simulink model "novel_topology_1"  (R2020a)
settings: Solver=FixedStepDiscrete  StartTime=0.0  StopTime=0.2  RelTol=1e-3
InitFcn:
  | novel_topology_1_param
values from neighbouring files (symbols this model uses):
  ar = 9    [novel_topology_1_param.m]    (also in novel_topology_2_param.m = 8)
libraries: powerlib_meascontrol x33, powerlib x31
settings Model: Creator=Raghuram  LastModifiedBy=Raghuram Shankar
settings DataIOCC: ReturnWorkspaceOutputs=off
settings OptimizationCC: LifeSpan=inf
settings DebuggingCC: SFExecutionAtInitializationDiag=none  ArithmeticOperatorsInVariantConditions=warning
settings SFSimCC: SimUseLocalCustomCode=off  CustomCodeUndefinedFunction=UseInterfaceOnly
settings RTWCC: RTWUseLocalCustomCode=off
settings CodeAppCC: StateflowObjectComments=on

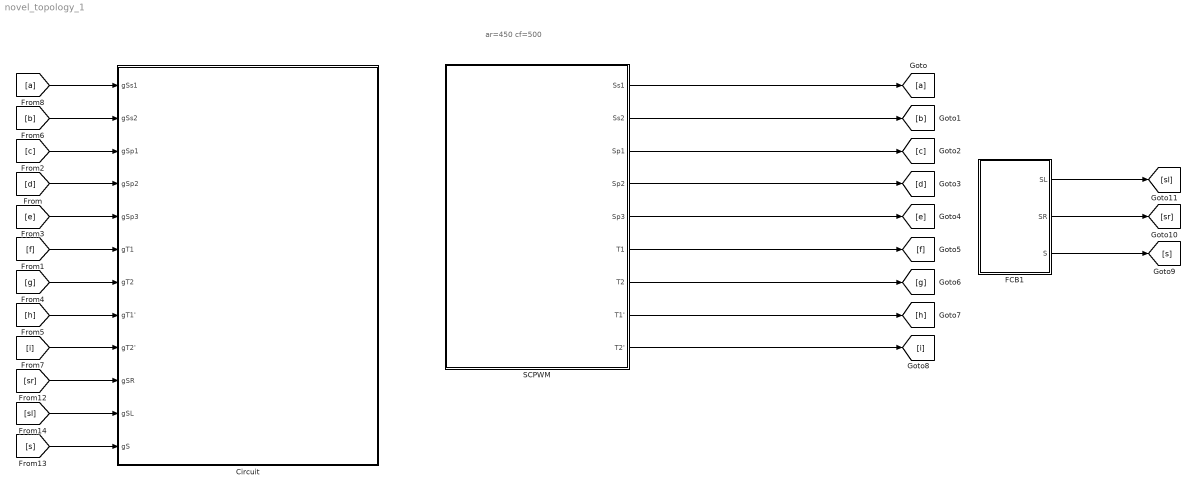
== system novel_topology_1 ==
  note: ar=450 cf=500
  Circuit : Subsystem
  FCB1 : Subsystem
  SCPWM : Subsystem
  wires:
  FCB1/1(SL) -> [sl]
  FCB1/3(S) -> [s]
  FCB1/2(SR) -> [sr]
  SCPWM/8(T1') -> [h]
  SCPWM/4(Sp2) -> [d]
  SCPWM/6(T1) -> [f]
  SCPWM/7(T2) -> [g]
  SCPWM/2(Ss2) -> [b]
  SCPWM/9(T2') -> [i]
  SCPWM/1(Ss1) -> [a]
  SCPWM/3(Sp1) -> [c]
  SCPWM/5(Sp3) -> [e]
  [a] -> Circuit/1(gSs1)
  [b] -> Circuit/2(gSs2)
  [c] -> Circuit/3(gSp1)
  [d] -> Circuit/4(gSp2)
  [e] -> Circuit/5(gSp3)
  [f] -> Circuit/6(gT1)
  [g] -> Circuit/7(gT2)
  [h] -> Circuit/8(gT1')
  [i] -> Circuit/9(gT2')
  [sr] -> Circuit/10(gSR)
  [sl] -> Circuit/11(gSL)
  [s] -> Circuit/12(gS)

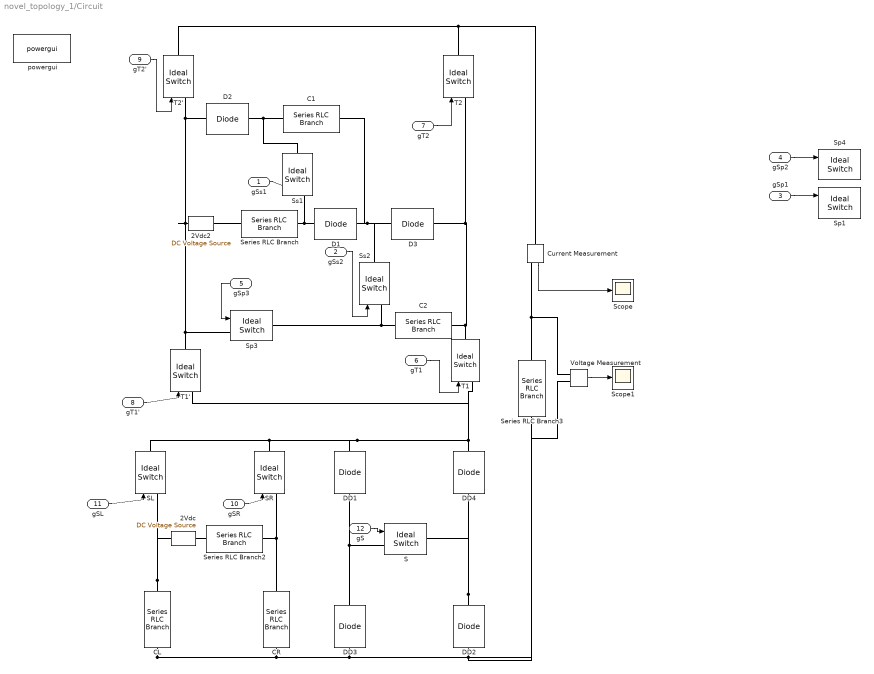
== system novel_topology_1/Circuit ==
  gSs1 : Inport
  gSs2 : Inport  Port=2
  gSp1 : Inport  Port=3
  gSp2 : Inport  Port=4
  gSp3 : Inport  Port=5
  gT1 : Inport  Port=6
  gT2 : Inport  Port=7
  gT1' : Inport  Port=8
  gT2' : Inport  Port=9
  gSR : Inport  Port=10
  gSL : Inport  Port=11
  gS : Inport  Port=12
  2Vdc : powerlib/Electrical Sources/DC Voltage Source  Amplitude=100  Measurements=None
  2Vdc2 : powerlib/Electrical Sources/DC Voltage Source  Amplitude=100  Measurements=None
  C1 : powerlib/Elements/Series RLC Branch  LConnTagsString=__new0  RConnTagsString=__new0  BranchType=C  Resistance=2.9e-3  Inductance=1e-3  SetiL0=off  InitialCurrent=0  Capacitance=2000e-6  Setx0=off  InitialVoltage=0  Measurements=None
  C2 : powerlib/Elements/Series RLC Branch  LConnTagsString=__new0  RConnTagsString=__new0  BranchType=C  Resistance=1.9e-3  Inductance=1e-3  SetiL0=off  InitialCurrent=0  Capacitance=3000e-6  Setx0=off  InitialVoltage=0  Measurements=None
  CL : powerlib/Elements/Series RLC Branch  LConnTagsString=__new0  RConnTagsString=__new0  BranchType=C  Resistance=3.9e-3  Inductance=1e-3  SetiL0=off  InitialCurrent=0  Capacitance=1000e-6  Setx0=off  InitialVoltage=0  Measurements=None
  CR : powerlib/Elements/Series RLC Branch  LConnTagsString=__new0  RConnTagsString=__new0  BranchType=C  Resistance=3.9e-3  Inductance=1e-3  SetiL0=off  InitialCurrent=0  Capacitance=1000e-6  Setx0=off  InitialVoltage=0  Measurements=None
  Current Measurement : powerlib/Measurements/Current Measurement  PhasorSimulation=off  OutputType=Complex  PSBequivalent=0
  D1 : powerlib/Power Electronics/Diode  Ron=0.1  Lon=0  Vf=1.06  IC=0  UseSnubber=0  Rs=10e8  Cs=10e-9  Measurements=off
  D2 : powerlib/Power Electronics/Diode  Ron=0.1  Lon=0  Vf=1.06  IC=0  UseSnubber=0  Rs=10e8  Cs=10e-9  Measurements=off
  D3 : powerlib/Power Electronics/Diode  Ron=0.1  Lon=0  Vf=1.06  IC=0  UseSnubber=0  Rs=10e8  Cs=10e-9  Measurements=off
  DD1 : powerlib/Power Electronics/Diode  Ron=0.2  Lon=0  Vf=1.06  IC=0  UseSnubber=0  Rs=10e8  Cs=10e-9  Measurements=off
  DD2 : powerlib/Power Electronics/Diode  Ron=0.2  Lon=0  Vf=1.06  IC=0  UseSnubber=0  Rs=10e8  Cs=10e-9  Measurements=off
  DD3 : powerlib/Power Electronics/Diode  Ron=0.2  Lon=0  Vf=1.06  IC=0  UseSnubber=0  Rs=10e8  Cs=10-9  Measurements=off
  DD4 : powerlib/Power Electronics/Diode  Ron=0.2  Lon=0  Vf=1.06  IC=0  UseSnubber=0  Rs=10e8  Cs=10e-9  Measurements=off
  S : powerlib/Power Electronics/Ideal Switch  Ron=0.001  Lon=0  IC=0  Rs=10e8  Cs=10e-9  Measurements=off
  SL : powerlib/Power Electronics/Ideal Switch  Ron=0.001  Lon=0  IC=0  Rs=10e8  Cs=10e-9  Measurements=off
  SR : powerlib/Power Electronics/Ideal Switch  Ron=0.001  Lon=0  IC=0  Rs=10e8  Cs=10e-9  Measurements=off
  Scope : Scope
  Scope1 : Scope
  Series RLC Branch : powerlib/Elements/Series RLC Branch  LConnTagsString=__new0  RConnTagsString=__new0  BranchType=R  Resistance=10e-9  Inductance=1e-3  SetiL0=off  InitialCurrent=0  Capacitance=1e-6  Setx0=off  InitialVoltage=0  Measurements=None
  Series RLC Branch2 : powerlib/Elements/Series RLC Branch  LConnTagsString=__new0  RConnTagsString=__new0  BranchType=R  Resistance=0.000001  Inductance=1e-3  SetiL0=off  InitialCurrent=0  Capacitance=1e-6  Setx0=off  InitialVoltage=0  Measurements=None
  Series RLC Branch3 : powerlib/Elements/Series RLC Branch  LConnTagsString=__new0  RConnTagsString=__new0  BranchType=R  Resistance=190  Inductance=200e-3  SetiL0=off  InitialCurrent=0  Capacitance=1e-6  Setx0=off  InitialVoltage=0  Measurements=None
  Sp1 : powerlib/Power Electronics/Ideal Switch  Ron=0.001  Lon=0  IC=0  Rs=10e8  Cs=10e-9  Measurements=off
  Sp3 : powerlib/Power Electronics/Ideal Switch  Ron=0.001  Lon=0  IC=0  Rs=10e8  Cs=10e-9  Measurements=off
  Sp4 : powerlib/Power Electronics/Ideal Switch  Ron=0.001  Lon=0  IC=0  Rs=10e8  Cs=10e-9  Measurements=off
  Ss1 : powerlib/Power Electronics/Ideal Switch  Ron=0.001  Lon=0  IC=0  Rs=10e8  Cs=10e-9  Measurements=off
  Ss2 : powerlib/Power Electronics/Ideal Switch  Ron=0.001  Lon=0  IC=0  Rs=10e8  Cs=10e-9  Measurements=off
  T1 : powerlib/Power Electronics/Ideal Switch  Ron=0.001  Lon=0  IC=0  Rs=10e8  Cs=10e-9  Measurements=off
  T1' : powerlib/Power Electronics/Ideal Switch  Ron=0.001  Lon=0  IC=0  Rs=10e8  Cs=10e-9  Measurements=off
  "T2 " : powerlib/Power Electronics/Ideal Switch  Ron=0.001  Lon=0  IC=0  Rs=10e8  Cs=10e-9  Measurements=off
  T2' : powerlib/Power Electronics/Ideal Switch  Ron=0.001  Lon=0  IC=0  Rs=10e8  Cs=10e-9  Measurements=off
  Voltage Measurement : powerlib/Measurements/Voltage Measurement  PhasorSimulation=off  OutputType=Complex  PSBequivalent=0
  powergui : powerlib/powergui  Priority=1  SimulationMode=Discrete  SampleTime=50e-6  frequency=60  Iterations=50  frequencyindice=0  Pbase=100e6  ErrMax=1e-4  UnitsV=kV  UnitsW=MW  buscounter=0  FunctionMessages=off  echomessages=off  EnableUseOfTLC=off  CurrentSourceSwitches=off  DisableSnubberDevices=off  DisableRonSwitches=off  DisableVfSwitches=off  DisplayEquations=off  AutomaticDiscreteSolvers=off  SolverType=Tustin/Backward Euler (TBE)  Interpol=off  ExternalGateDelay=off  methode=off  Ts=100  x0status=blocks  SPID=on  SwTol=0  HookPort=off  NonlinearTolerance=1e-4  nMaxIteration=100  ContinueOnMaxIteration=off  RestoreLinks=warning  ResistiveCurrentMeasurement=off  Frange=[0:2:500]  Ylog=off  Xlog=on  ShowGrid=off  save=off  variable=ZData  structure=novel1cur  ZoomFFT=off  StartTime=0.04  cycles=8  DisplayStyle=1  fundamental=50  FreqAxis=on  MaxFrequency=1000  frequencyindicesteady=1  RmsSteady=1  display=off
  wires:
  Current Measurement/1 -> Scope/1
  gSp1/1 -> Sp1/1
  gT2/1 -> "T2 "/1
  gSs2/1 -> Ss2/1
  gSs1/1 -> Ss1/1
  gT1'/1 -> T1'/1
  gT1/1 -> T1/1
  gT2'/1 -> T2'/1
  gSp3/1 -> Sp3/1
  gSL/1 -> SL/1
  gS/1 -> S/1
  gSR/1 -> SR/1
  gSp2/1 -> Sp4/1
  Voltage Measurement/1 -> Scope1/1
  connections:
  Ss1/LConn1 -- Series RLC Branch/RConn1 -- D1/LConn1
  Ss2/LConn1 -- Sp3/RConn1 -- C2/RConn1
  DD2/LConn1 -- S/RConn1 -- DD4/LConn1
  DD3/RConn1 -- S/LConn1 -- DD1/RConn1
  CL/LConn1 -- 2Vdc/RConn1 -- SL/LConn1
  SR/LConn1 -- CR/RConn1 -- Series RLC Branch2/LConn1
  CL/RConn1 -- CR/LConn1 -- Voltage Measurement/LConn2 -- Series RLC Branch3/RConn1 -- DD2/RConn1 -- DD3/LConn1
  2Vdc/LConn1 -- Series RLC Branch2/RConn1
  2Vdc2/RConn1 -- Series RLC Branch/LConn1
  T2'/RConn1 -- Current Measurement/LConn1 -- "T2 "/RConn1
  SL/RConn1 -- T1'/LConn1 -- T1/LConn1 -- DD4/RConn1 -- DD1/LConn1 -- SR/RConn1
  T2'/LConn1 -- D2/RConn1 -- Sp3/LConn1 -- T1'/RConn1 -- 2Vdc2/LConn1
  "T2 "/LConn1 -- D3/RConn1 -- C2/LConn1 -- T1/RConn1
  C1/LConn1 -- D3/LConn1 -- Ss2/RConn1 -- D1/RConn1
  D2/LConn1 -- Ss1/RConn1 -- C1/RConn1
  Current Measurement/RConn1 -- Voltage Measurement/LConn1 -- Series RLC Branch3/LConn1

== system novel_topology_1/FCB1 ==
  Logical Operator : Logic  Operator=NOR  AllPortsSameDT=off  OutDataTypeStr=boolean
  PWMSL : Subsystem
  PWMSR : Subsystem
  Scope : Scope
  Scope1 : Scope
  Scope2 : Scope
  SL : Outport  VectorParamsAs1DForOutWhenUnconnected=off
  SR : Outport  Port=2  VectorParamsAs1DForOutWhenUnconnected=off
  S : Outport  Port=3  VectorParamsAs1DForOutWhenUnconnected=off
  wires:
  Logical Operator/1 -> Scope2/1, S/1
  PWMSL/1(SL) -> Scope/1, SL/1, Logical Operator/2
  PWMSR/1(SR) -> Logical Operator/1, Scope1/1, SR/1

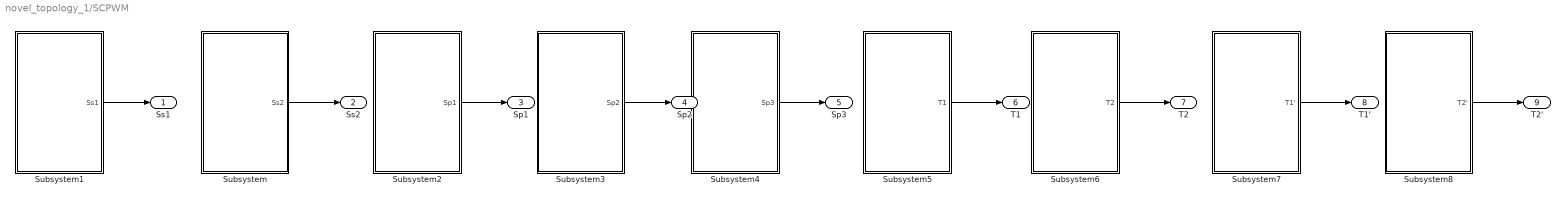
== system novel_topology_1/SCPWM ==
  Subsystem : Subsystem
  Subsystem1 : Subsystem
  Subsystem2 : Subsystem
  Subsystem3 : Subsystem
  Subsystem4 : Subsystem
  Subsystem5 : Subsystem
  Subsystem6 : Subsystem
  Subsystem7 : Subsystem
  Subsystem8 : Subsystem
  Ss1 : Outport  VectorParamsAs1DForOutWhenUnconnected=off
  Ss2 : Outport  Port=2  VectorParamsAs1DForOutWhenUnconnected=off
  Sp1 : Outport  Port=3  VectorParamsAs1DForOutWhenUnconnected=off
  Sp2 : Outport  Port=4  VectorParamsAs1DForOutWhenUnconnected=off
  Sp3 : Outport  Port=5  VectorParamsAs1DForOutWhenUnconnected=off
  T1 : Outport  Port=6  VectorParamsAs1DForOutWhenUnconnected=off
  T2 : Outport  Port=7  VectorParamsAs1DForOutWhenUnconnected=off
  T1' : Outport  Port=8  VectorParamsAs1DForOutWhenUnconnected=off
  T2' : Outport  Port=9  VectorParamsAs1DForOutWhenUnconnected=off
  wires:
  Subsystem7/1(T1') -> T1'/1
  Subsystem/1(Ss2) -> Ss2/1
  Subsystem3/1(Sp2) -> Sp2/1
  Subsystem6/1(T2) -> T2/1
  Subsystem2/1(Sp1) -> Sp1/1
  Subsystem5/1(T1) -> T1/1
  Subsystem8/1(T2') -> T2'/1
  Subsystem4/1(Sp3) -> Sp3/1
  Subsystem1/1(Ss1) -> Ss1/1

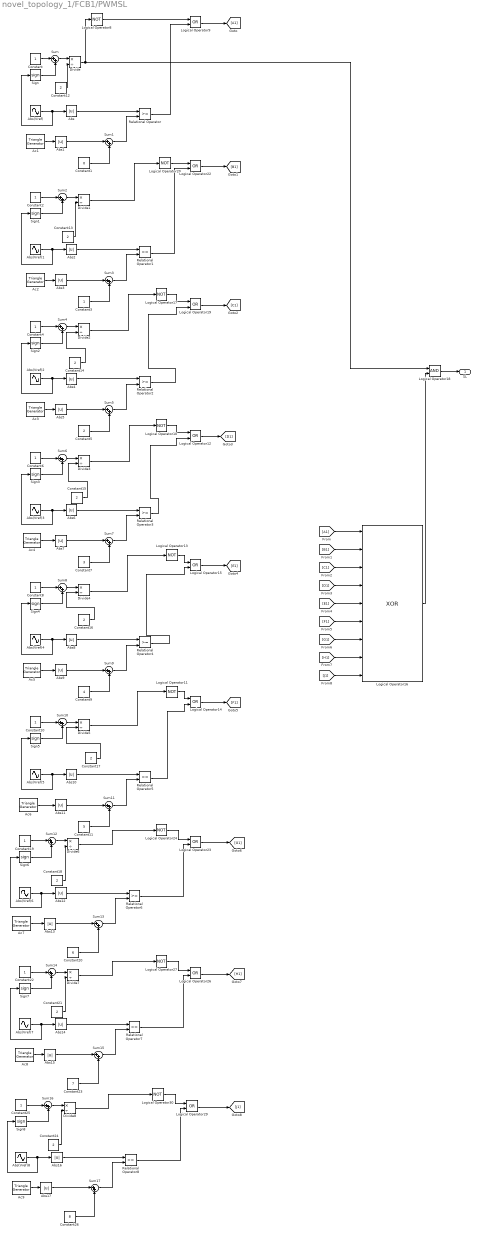
== system novel_topology_1/FCB1/PWMSL ==
  Abs{,1..17} (18 alike) : Abs
  Abs(Vref){,1..8} (9 alike) : Sin  Amplitude=ar  Frequency=2*pi*50  SampleTime=0
  Ac1 : powerlib_meascontrol/Pulse & Signal Generators/Triangle Generator  Freq=cf  Phase=0  Ts=0
  Ac{2..6,8..9} (7 alike) : powerlib_meascontrol/Pulse & Signal Generators/Triangle Generator  Freq=cf  Phase=90  Ts=0
  "Ac7 " : powerlib_meascontrol/Pulse & Signal Generators/Triangle Generator  Freq=cf  Phase=90  Ts=0
  Constant{,2..4,6,8,10,19,22,25} (10 alike) : Constant
  Constant1 : Constant  Value=0
  Constant11 : Constant  Value=5
  Constant{5,12..18,21,24} (10 alike) : Constant  Value=2
  Constant20 : Constant  Value=6
  Constant23 : Constant  Value=7
  Constant26 : Constant  Value=8
  Constant7 : Constant  Value=3
  Constant9 : Constant  Value=4
  Divide{,1..8} (9 alike) : Product  Inputs=*/
  Logical Operator{8,10..11,13,17,20,24,27,30} (9 alike) : Logic  Operator=NOT  AllPortsSameDT=off  OutDataTypeStr=boolean
  Logical Operator{9,12,14..15,19,22..23,26,29} (9 alike) : Logic  Operator=OR  AllPortsSameDT=off  OutDataTypeStr=boolean
  Logical Operator16 : Logic  Operator=XOR  Inputs=9  AllPortsSameDT=off  OutDataTypeStr=boolean
  Logical Operator18 : Logic  AllPortsSameDT=off  OutDataTypeStr=boolean
  Relational Operator{,1..8} (9 alike) : RelationalOperator  OutDataTypeStr=boolean  RndMeth=Nearest
  Sign{,1..8} (9 alike) : Signum
  Sum{,1..17} (18 alike) : Sum  Inputs=|++
  SL : Outport  VectorParamsAs1DForOutWhenUnconnected=off
  wires:
  Abs1/1 -> Sum1/1
  Divide5/1 -> Logical Operator11/1
  Sum2/1 -> Divide1/1
  Abs5/1 -> Sum5/1
  Sum8/1 -> Divide4/1
  Relational Operator3/1 -> Logical Operator12/2
  Abs(Vref)4/1 -> Sign4/1, Abs8/1
  Divide4/1 -> Logical Operator13/1
  Abs(Vref)/1 -> Sign/1, Abs/1
  Logical Operator11/1 -> Logical Operator14/1
  Constant/1 -> Sum/1
  Relational Operator1/1 -> Logical Operator22/2
  Sum11/1 -> Relational Operator5/2
  Sum/1 -> Divide/1
  Abs2/1 -> Relational Operator1/1
  Divide3/1 -> Logical Operator10/1
  Divide1/1 -> Logical Operator20/1
  Abs8/1 -> Relational Operator4/1
  Abs(Vref)1/1 -> Sign1/1, Abs2/1
  Sign3/1 -> Sum6/2
  Relational Operator/1 -> Logical Operator9/2
  Abs(Vref)2/1 -> Sign2/1, Abs4/1
  Abs6/1 -> Relational Operator3/1
  Abs(Vref)3/1 -> Sign3/1, Abs6/1
  Logical Operator17/1 -> Logical Operator19/1
  Sign2/1 -> Sum4/2
  Divide/1 -> Logical Operator18/1, Logical Operator8/1
  Logical Operator18/1 -> SL/1
  Sum7/1 -> Relational Operator3/2
  Sign1/1 -> Sum2/2
  Sum4/1 -> Divide2/1
  Sum1/1 -> Relational Operator/2
  Constant2/1 -> Sum2/1
  Divide2/1 -> Logical Operator17/1
  Sign4/1 -> Sum8/2
  Abs10/1 -> Relational Operator5/1
  Constant13/1 -> Divide1/2
  Constant11/1 -> Sum11/2
  Abs/1 -> Relational Operator/1
  Constant3/1 -> Sum3/2
  Constant4/1 -> Sum4/1
  Abs(Vref)5/1 -> Sign5/1, Abs10/1
  Logical Operator20/1 -> Logical Operator22/1
  Constant17/1 -> Divide5/2
  Constant10/1 -> Sum10/1
  Constant1/1 -> Sum1/2
  Constant6/1 -> Sum6/1
  Abs11/1 -> Sum11/1
  Logical Operator16/1 -> Logical Operator18/2
  Logical Operator8/1 -> Logical Operator9/1
  Constant9/1 -> Sum9/2
  Abs9/1 -> Sum9/1
  Logical Operator10/1 -> Logical Operator12/1
  Relational Operator2/1 -> Logical Operator19/2
  Relational Operator5/1 -> Logical Operator14/2
  Relational Operator4/1 -> Logical Operator15/2
  Constant15/1 -> Divide3/2
  Constant16/1 -> Divide4/2
  Constant12/1 -> Divide/2
  Constant14/1 -> Divide2/2
  Logical Operator13/1 -> Logical Operator15/1
  Abs4/1 -> Relational Operator2/1
  Sum9/1 -> Relational Operator4/2
  Constant7/1 -> Sum7/2
  Constant5/1 -> Sum5/2
  Sum5/1 -> Relational Operator2/2
  Constant8/1 -> Sum8/1
  Sign/1 -> Sum/2
  Abs3/1 -> Sum3/1
  Abs7/1 -> Sum7/1
  Sum3/1 -> Relational Operator1/2
  Sign5/1 -> Sum10/2
  Sum6/1 -> Divide3/1
  Sum10/1 -> Divide5/1
  Divide6/1 -> Logical Operator24/1
  Constant19/1 -> Sum12/1
  Constant18/1 -> Divide6/2
  Abs(Vref)6/1 -> Sign6/1, Abs12/1
  Relational Operator6/1 -> Logical Operator23/2
  Abs12/1 -> Relational Operator6/1
  Abs13/1 -> Sum13/1
  Sum12/1 -> Divide6/1
  Sum13/1 -> Relational Operator6/2
  Sign6/1 -> Sum12/2
  Constant20/1 -> Sum13/2
  Logical Operator24/1 -> Logical Operator23/1
  Logical Operator27/1 -> Logical Operator26/1
  Constant22/1 -> Sum14/1
  Sum15/1 -> Relational Operator7/2
  Abs15/1 -> Sum15/1
  Sum14/1 -> Divide7/1
  Abs14/1 -> Relational Operator7/1
  Constant23/1 -> Sum15/2
  Abs(Vref)7/1 -> Sign7/1, Abs14/1
  Divide7/1 -> Logical Operator27/1
  Sign7/1 -> Sum14/2
  Constant21/1 -> Divide7/2
  Relational Operator7/1 -> Logical Operator26/2
  Logical Operator30/1 -> Logical Operator29/1
  Constant25/1 -> Sum16/1
  Sum17/1 -> Relational Operator8/2
  Abs17/1 -> Sum17/1
  Sum16/1 -> Divide8/1
  Abs16/1 -> Relational Operator8/1
  Constant26/1 -> Sum17/2
  Abs(Vref)8/1 -> Sign8/1, Abs16/1
  Divide8/1 -> Logical Operator30/1
  Sign8/1 -> Sum16/2
  Constant24/1 -> Divide8/2
  Relational Operator8/1 -> Logical Operator29/2
  [A1] -> Logical Operator16/1
  [B1] -> Logical Operator16/2
  [C1] -> Logical Operator16/3
  [D1] -> Logical Operator16/4
  [E1] -> Logical Operator16/5
  [F1] -> Logical Operator16/6
  [G1] -> Logical Operator16/7
  [H1] -> Logical Operator16/8
  Ac1/1 -> Abs1/1
  Ac2/1 -> Abs3/1
  Ac3/1 -> Abs5/1
  Ac4/1 -> Abs7/1
  Ac5/1 -> Abs9/1
  Ac6/1 -> Abs11/1
  Ac9/1 -> Abs17/1
  "Ac7 "/1 -> Abs13/1
  Ac8/1 -> Abs15/1
  Logical Operator22/1 -> [B1]
  Logical Operator19/1 -> [C1]
  Logical Operator12/1 -> [D1]
  Logical Operator15/1 -> [E1]
  Logical Operator14/1 -> [F1]
  Logical Operator23/1 -> [G1]
  Logical Operator26/1 -> [H1]
  Logical Operator29/1 -> [J1]
  [J1] -> Logical Operator16/9
  Logical Operator9/1 -> [A1]

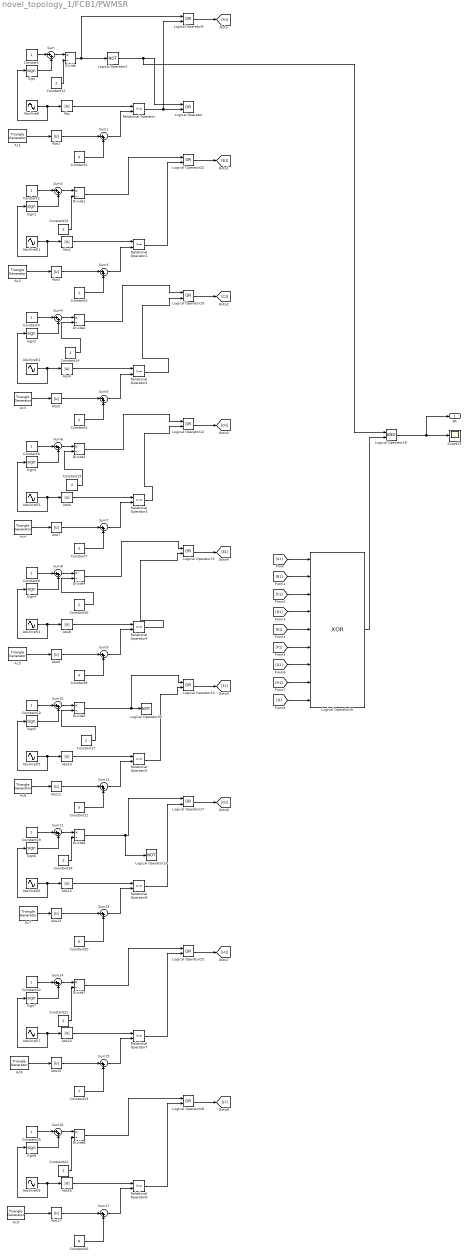
== system novel_topology_1/FCB1/PWMSR ==
  Abs{,1..17} (18 alike) : Abs
  Abs(Vref){,1..8} (9 alike) : Sin  Amplitude=ar  Frequency=2*pi*50  SampleTime=0
  Ac1 : powerlib_meascontrol/Pulse & Signal Generators/Triangle Generator  Freq=cf  Phase=0  Ts=0
  Ac{2..9} (8 alike) : powerlib_meascontrol/Pulse & Signal Generators/Triangle Generator  Freq=cf  Phase=90  Ts=0
  Constant{,2..4,6,8,10,19,22,25} (10 alike) : Constant
  Constant1 : Constant  Value=0
  Constant11 : Constant  Value=5
  Constant{5,12..18,21,24} (10 alike) : Constant  Value=2
  Constant20 : Constant  Value=6
  Constant23 : Constant  Value=7
  Constant26 : Constant  Value=8
  Constant7 : Constant  Value=3
  Constant9 : Constant  Value=4
  Divide{,1..8} (9 alike) : Product  Inputs=*/
  Logical Operator{,9,12,14..15,17,19,22,25,28} (10 alike) : Logic  Operator=OR  AllPortsSameDT=off  OutDataTypeStr=boolean
  Logical Operator13 : Logic  Operator=NOT  AllPortsSameDT=off  OutDataTypeStr=boolean
  Logical Operator16 : Logic  Operator=XOR  Inputs=9  AllPortsSameDT=off  OutDataTypeStr=boolean
  Logical Operator18 : Logic  AllPortsSameDT=off  OutDataTypeStr=boolean
  Logical Operator2 : Logic  Operator=NOT  AllPortsSameDT=off  OutDataTypeStr=boolean
  Logical Operator30 : Logic  Operator=NOT  AllPortsSameDT=off  OutDataTypeStr=boolean
  Relational Operator{,1..8} (9 alike) : RelationalOperator  OutDataTypeStr=boolean  RndMeth=Nearest
  Scope13 : Scope
  Sign{,1..8} (9 alike) : Signum
  Sum{,1..17} (18 alike) : Sum  Inputs=|++
  SR : Outport  VectorParamsAs1DForOutWhenUnconnected=off
  wires:
  Abs1/1 -> Sum1/1
  Sum2/1 -> Divide1/1
  Abs5/1 -> Sum5/1
  Sum8/1 -> Divide4/1
  Relational Operator3/1 -> Logical Operator12/2
  Abs(Vref)4/1 -> Sign4/1, Abs8/1
  Abs(Vref)/1 -> Sign/1, Abs/1
  Divide5/1 -> Logical Operator30/1, Logical Operator14/1
  Constant/1 -> Sum/1
  Relational Operator1/1 -> Logical Operator22/2
  Sum11/1 -> Relational Operator5/2
  Sum/1 -> Divide/1
  Abs2/1 -> Relational Operator1/1
  Abs8/1 -> Relational Operator4/1
  Abs(Vref)1/1 -> Sign1/1, Abs2/1
  Sign3/1 -> Sum6/2
  Relational Operator/1 -> Logical Operator9/2, Logical Operator/2
  Abs(Vref)2/1 -> Sign2/1, Abs4/1
  Abs6/1 -> Relational Operator3/1
  Abs(Vref)3/1 -> Sign3/1, Abs6/1
  Divide2/1 -> Logical Operator19/1
  Sign2/1 -> Sum4/2
  Logical Operator18/1 -> SR/1, Scope13/1
  Sum7/1 -> Relational Operator3/2
  Sign1/1 -> Sum2/2
  Sum4/1 -> Divide2/1
  Sum1/1 -> Relational Operator/2
  Constant2/1 -> Sum2/1
  Sign4/1 -> Sum8/2
  Abs10/1 -> Relational Operator5/1
  Constant13/1 -> Divide1/2
  Constant11/1 -> Sum11/2
  Abs/1 -> Relational Operator/1
  Constant3/1 -> Sum3/2
  Constant4/1 -> Sum4/1
  Abs(Vref)5/1 -> Sign5/1, Abs10/1
  Divide1/1 -> Logical Operator22/1
  Constant17/1 -> Divide5/2
  Constant10/1 -> Sum10/1
  Constant1/1 -> Sum1/2
  Constant6/1 -> Sum6/1
  Abs11/1 -> Sum11/1
  Logical Operator16/1 -> Logical Operator18/2
  Divide/1 -> Logical Operator9/1, Logical Operator2/1
  Constant9/1 -> Sum9/2
  Abs9/1 -> Sum9/1
  Divide3/1 -> Logical Operator12/1
  Relational Operator2/1 -> Logical Operator19/2
  Relational Operator5/1 -> Logical Operator14/2
  Relational Operator4/1 -> Logical Operator15/2
  Constant15/1 -> Divide3/2
  Constant16/1 -> Divide4/2
  Constant12/1 -> Divide/2
  Constant14/1 -> Divide2/2
  Divide4/1 -> Logical Operator15/1
  Abs4/1 -> Relational Operator2/1
  Sum9/1 -> Relational Operator4/2
  Constant7/1 -> Sum7/2
  Constant5/1 -> Sum5/2
  Sum5/1 -> Relational Operator2/2
  Constant8/1 -> Sum8/1
  Sign/1 -> Sum/2
  Abs3/1 -> Sum3/1
  Abs7/1 -> Sum7/1
  Sum3/1 -> Relational Operator1/2
  Sign5/1 -> Sum10/2
  Sum6/1 -> Divide3/1
  Sum10/1 -> Divide5/1
  Logical Operator2/1 -> Logical Operator18/1, Logical Operator/1
  Constant19/1 -> Sum12/1
  Constant18/1 -> Divide6/2
  Abs(Vref)6/1 -> Sign6/1, Abs12/1
  Relational Operator6/1 -> Logical Operator17/2
  Abs12/1 -> Relational Operator6/1
  Abs13/1 -> Sum13/1
  Sum12/1 -> Divide6/1
  Divide6/1 -> Logical Operator17/1, Logical Operator13/1
  Sum13/1 -> Relational Operator6/2
  Sign6/1 -> Sum12/2
  Constant20/1 -> Sum13/2
  Sum15/1 -> Relational Operator7/2
  Relational Operator7/1 -> Logical Operator25/2
  Sum14/1 -> Divide7/1
  Constant23/1 -> Sum15/2
  Abs15/1 -> Sum15/1
  Abs(Vref)7/1 -> Sign7/1, Abs14/1
  Sign7/1 -> Sum14/2
  Abs14/1 -> Relational Operator7/1
  Constant21/1 -> Divide7/2
  Divide7/1 -> Logical Operator25/1
  Constant22/1 -> Sum14/1
  Sum17/1 -> Relational Operator8/2
  Relational Operator8/1 -> Logical Operator28/2
  Sum16/1 -> Divide8/1
  Constant26/1 -> Sum17/2
  Abs17/1 -> Sum17/1
  Abs(Vref)8/1 -> Sign8/1, Abs16/1
  Sign8/1 -> Sum16/2
  Abs16/1 -> Relational Operator8/1
  Constant24/1 -> Divide8/2
  Divide8/1 -> Logical Operator28/1
  Constant25/1 -> Sum16/1
  [E1] -> Logical Operator16/5
  [D1] -> Logical Operator16/4
  [B1] -> Logical Operator16/2
  [F1] -> Logical Operator16/6
  [A1] -> Logical Operator16/1
  [G1] -> Logical Operator16/7
  [H1] -> Logical Operator16/8
  [C1] -> Logical Operator16/3
  Ac1/1 -> Abs1/1
  Ac2/1 -> Abs3/1
  Ac3/1 -> Abs5/1
  Ac4/1 -> Abs7/1
  Ac8/1 -> Abs15/1
  Ac9/1 -> Abs17/1
  Ac7/1 -> Abs13/1
  Ac6/1 -> Abs11/1
  Ac5/1 -> Abs9/1
  Logical Operator9/1 -> [A1]
  Logical Operator22/1 -> [B1]
  Logical Operator19/1 -> [C1]
  Logical Operator12/1 -> [D1]
  Logical Operator15/1 -> [E1]
  Logical Operator14/1 -> [F1]
  Logical Operator17/1 -> [G1]
  Logical Operator25/1 -> [H1]
  Logical Operator28/1 -> [J1]
  [J1] -> Logical Operator16/9

== system novel_topology_1/SCPWM/Subsystem ==
  Abs : Abs
  Abs(Vref) : Sin  Amplitude=ar  Frequency=2*pi*50  SampleTime=0
  Abs1 : Abs
  Ac4 : powerlib_meascontrol/Pulse & Signal Generators/Triangle Generator  Freq=cf  Phase=90  Ts=0
  Constant1 : Constant  Value=5
  Relational Operator : RelationalOperator  OutDataTypeStr=boolean  RndMeth=Nearest
  Sum1 : Sum  Inputs=|++
  Ss2 : Outport  VectorParamsAs1DForOutWhenUnconnected=off
  wires:
  Abs/1 -> Relational Operator/1
  Abs(Vref)/1 -> Abs/1
  Ac4/1 -> Abs1/1
  Sum1/1 -> Relational Operator/2
  Abs1/1 -> Sum1/1
  Constant1/1 -> Sum1/2
  Relational Operator/1 -> Ss2/1

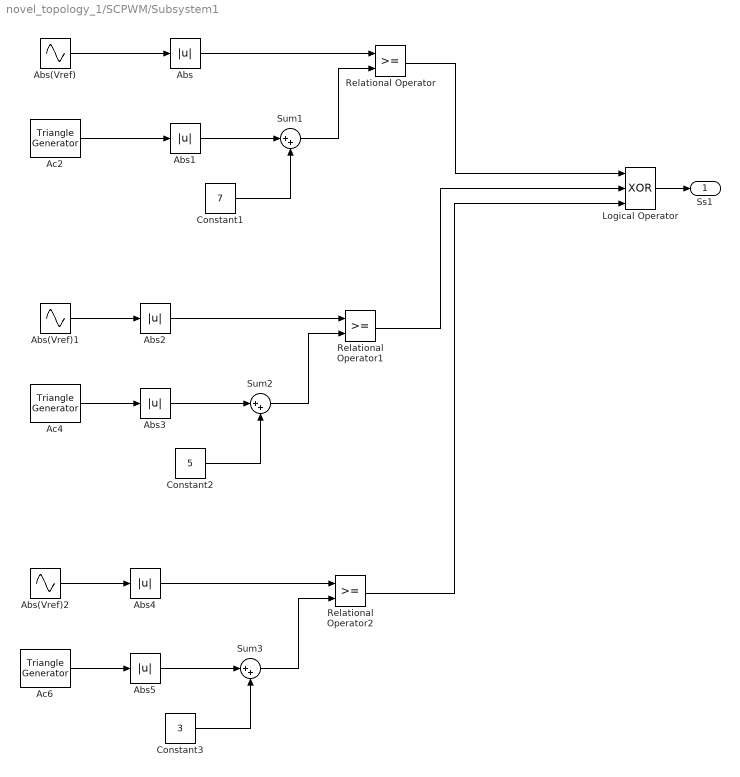
== system novel_topology_1/SCPWM/Subsystem1 ==
  Abs{,1..5} (6 alike) : Abs
  Abs(Vref) : Sin  Amplitude=ar  Frequency=2*pi*50  SampleTime=0
  Abs(Vref)1 : Sin  Amplitude=ar  Frequency=2*pi*50  SampleTime=0
  Abs(Vref)2 : Sin  Amplitude=ar  Frequency=2*pi*50  SampleTime=0
  Ac2 : powerlib_meascontrol/Pulse & Signal Generators/Triangle Generator  Freq=cf  Phase=90  Ts=0
  Ac4 : powerlib_meascontrol/Pulse & Signal Generators/Triangle Generator  Freq=cf  Phase=90  Ts=0
  Ac6 : powerlib_meascontrol/Pulse & Signal Generators/Triangle Generator  Freq=cf  Phase=90  Ts=0
  Constant1 : Constant  Value=7
  Constant2 : Constant  Value=5
  Constant3 : Constant  Value=3
  Logical Operator : Logic  Operator=XOR  Inputs=3  AllPortsSameDT=off  OutDataTypeStr=boolean
  Relational Operator : RelationalOperator  OutDataTypeStr=boolean  RndMeth=Nearest
  Relational Operator1 : RelationalOperator  OutDataTypeStr=boolean  RndMeth=Nearest
  Relational Operator2 : RelationalOperator  OutDataTypeStr=boolean  RndMeth=Nearest
  Sum1 : Sum  Inputs=|++
  Sum2 : Sum  Inputs=|++
  Sum3 : Sum  Inputs=|++
  Ss1 : Outport  VectorParamsAs1DForOutWhenUnconnected=off
  wires:
  Abs/1 -> Relational Operator/1
  Abs(Vref)/1 -> Abs/1
  Ac2/1 -> Abs1/1
  Sum1/1 -> Relational Operator/2
  Abs1/1 -> Sum1/1
  Constant1/1 -> Sum1/2
  Relational Operator/1 -> Logical Operator/1
  Sum2/1 -> Relational Operator1/2
  Ac4/1 -> Abs3/1
  Constant2/1 -> Sum2/2
  Abs3/1 -> Sum2/1
  Abs(Vref)1/1 -> Abs2/1
  Abs2/1 -> Relational Operator1/1
  Abs(Vref)2/1 -> Abs4/1
  Abs4/1 -> Relational Operator2/1
  Constant3/1 -> Sum3/2
  Abs5/1 -> Sum3/1
  Ac6/1 -> Abs5/1
  Sum3/1 -> Relational Operator2/2
  Relational Operator2/1 -> Logical Operator/3
  Relational Operator1/1 -> Logical Operator/2
  Logical Operator/1 -> Ss1/1

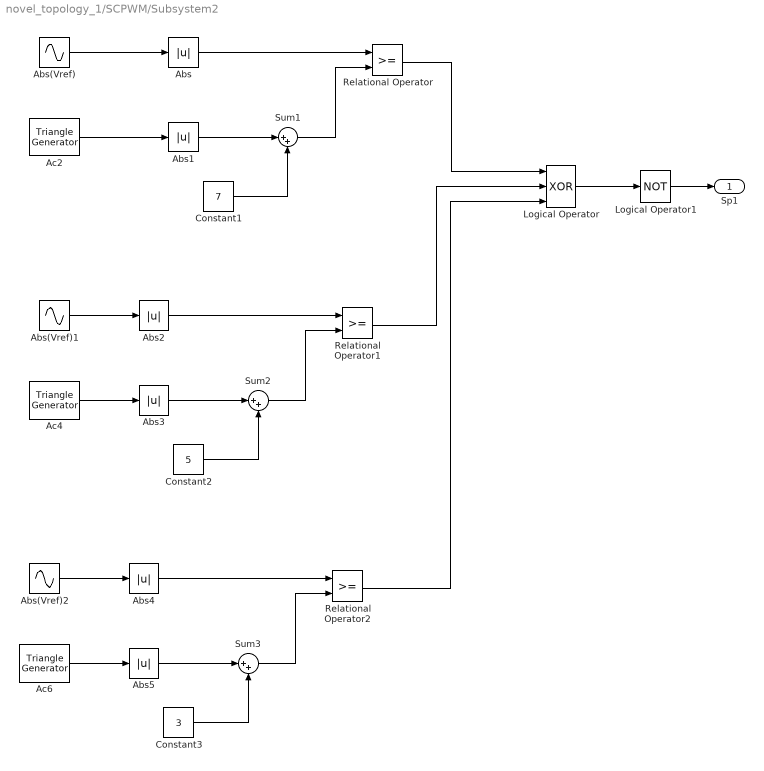
== system novel_topology_1/SCPWM/Subsystem2 ==
  Abs{,1..5} (6 alike) : Abs
  Abs(Vref) : Sin  Amplitude=ar  Frequency=2*pi*50  SampleTime=0
  Abs(Vref)1 : Sin  Amplitude=ar  Frequency=2*pi*50  SampleTime=0
  Abs(Vref)2 : Sin  Amplitude=ar  Frequency=2*pi*50  SampleTime=0
  Ac2 : powerlib_meascontrol/Pulse & Signal Generators/Triangle Generator  Freq=cf  Phase=90  Ts=0
  Ac4 : powerlib_meascontrol/Pulse & Signal Generators/Triangle Generator  Freq=cf  Phase=90  Ts=0
  Ac6 : powerlib_meascontrol/Pulse & Signal Generators/Triangle Generator  Freq=cf  Phase=90  Ts=0
  Constant1 : Constant  Value=7
  Constant2 : Constant  Value=5
  Constant3 : Constant  Value=3
  Logical Operator : Logic  Operator=XOR  Inputs=3  AllPortsSameDT=off  OutDataTypeStr=boolean
  Logical Operator1 : Logic  Operator=NOT  AllPortsSameDT=off  OutDataTypeStr=boolean
  Relational Operator : RelationalOperator  OutDataTypeStr=boolean  RndMeth=Nearest
  Relational Operator1 : RelationalOperator  OutDataTypeStr=boolean  RndMeth=Nearest
  Relational Operator2 : RelationalOperator  OutDataTypeStr=boolean  RndMeth=Nearest
  Sum1 : Sum  Inputs=|++
  Sum2 : Sum  Inputs=|++
  Sum3 : Sum  Inputs=|++
  Sp1 : Outport  VectorParamsAs1DForOutWhenUnconnected=off
  wires:
  Abs/1 -> Relational Operator/1
  Abs(Vref)/1 -> Abs/1
  Ac2/1 -> Abs1/1
  Sum1/1 -> Relational Operator/2
  Abs1/1 -> Sum1/1
  Constant1/1 -> Sum1/2
  Relational Operator/1 -> Logical Operator/1
  Sum2/1 -> Relational Operator1/2
  Ac4/1 -> Abs3/1
  Constant2/1 -> Sum2/2
  Abs3/1 -> Sum2/1
  Abs(Vref)1/1 -> Abs2/1
  Abs2/1 -> Relational Operator1/1
  Abs(Vref)2/1 -> Abs4/1
  Abs4/1 -> Relational Operator2/1
  Constant3/1 -> Sum3/2
  Abs5/1 -> Sum3/1
  Ac6/1 -> Abs5/1
  Sum3/1 -> Relational Operator2/2
  Relational Operator2/1 -> Logical Operator/3
  Relational Operator1/1 -> Logical Operator/2
  Logical Operator/1 -> Logical Operator1/1
  Logical Operator1/1 -> Sp1/1

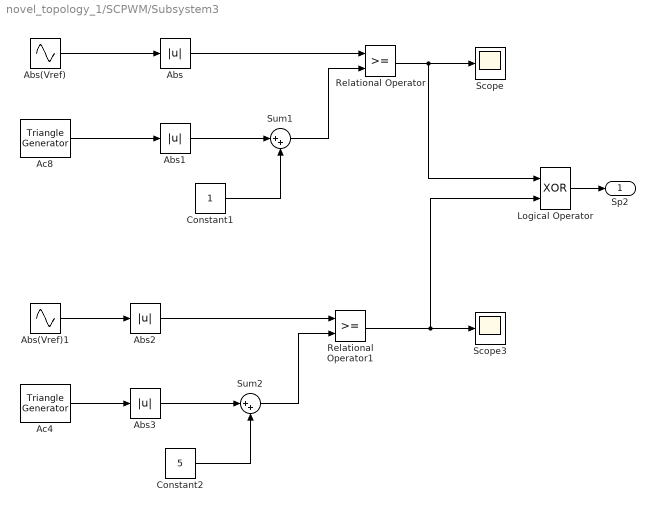
== system novel_topology_1/SCPWM/Subsystem3 ==
  Abs{,1..3} (4 alike) : Abs
  Abs(Vref) : Sin  Amplitude=ar  Frequency=2*pi*50  SampleTime=0
  Abs(Vref)1 : Sin  Amplitude=ar  Frequency=2*pi*50  SampleTime=0
  Ac4 : powerlib_meascontrol/Pulse & Signal Generators/Triangle Generator  Freq=cf  Phase=90  Ts=0
  Ac8 : powerlib_meascontrol/Pulse & Signal Generators/Triangle Generator  Freq=cf  Phase=90  Ts=0
  Constant1 : Constant
  Constant2 : Constant  Value=5
  Logical Operator : Logic  Operator=XOR  AllPortsSameDT=off  OutDataTypeStr=boolean
  Relational Operator : RelationalOperator  OutDataTypeStr=boolean  RndMeth=Nearest
  Relational Operator1 : RelationalOperator  OutDataTypeStr=boolean  RndMeth=Nearest
  Scope : Scope
  Scope3 : Scope
  Sum1 : Sum  Inputs=|++
  Sum2 : Sum  Inputs=|++
  Sp2 : Outport  VectorParamsAs1DForOutWhenUnconnected=off
  wires:
  Abs/1 -> Relational Operator/1
  Abs(Vref)/1 -> Abs/1
  Ac8/1 -> Abs1/1
  Sum1/1 -> Relational Operator/2
  Abs1/1 -> Sum1/1
  Constant1/1 -> Sum1/2
  Relational Operator/1 -> Scope/1, Logical Operator/1
  Sum2/1 -> Relational Operator1/2
  Ac4/1 -> Abs3/1
  Constant2/1 -> Sum2/2
  Abs3/1 -> Sum2/1
  Abs(Vref)1/1 -> Abs2/1
  Abs2/1 -> Relational Operator1/1
  Relational Operator1/1 -> Logical Operator/2, Scope3/1
  Logical Operator/1 -> Sp2/1

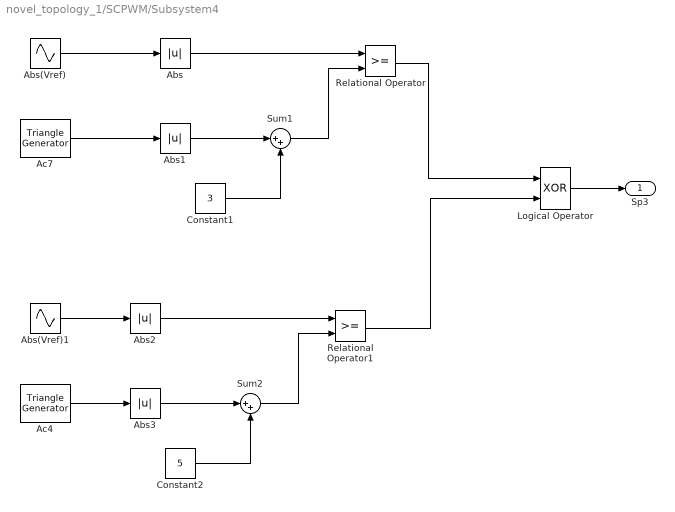
== system novel_topology_1/SCPWM/Subsystem4 ==
  Abs{,1..3} (4 alike) : Abs
  Abs(Vref) : Sin  Amplitude=ar  Frequency=2*pi*50  SampleTime=0
  Abs(Vref)1 : Sin  Amplitude=ar  Frequency=2*pi*50  SampleTime=0
  Ac4 : powerlib_meascontrol/Pulse & Signal Generators/Triangle Generator  Freq=cf  Phase=90  Ts=0
  Ac7 : powerlib_meascontrol/Pulse & Signal Generators/Triangle Generator  Freq=cf  Phase=90  Ts=0
  Constant1 : Constant  Value=3
  Constant2 : Constant  Value=5
  Logical Operator : Logic  Operator=XOR  AllPortsSameDT=off  OutDataTypeStr=boolean
  Relational Operator : RelationalOperator  OutDataTypeStr=boolean  RndMeth=Nearest
  Relational Operator1 : RelationalOperator  OutDataTypeStr=boolean  RndMeth=Nearest
  Sum1 : Sum  Inputs=|++
  Sum2 : Sum  Inputs=|++
  Sp3 : Outport  VectorParamsAs1DForOutWhenUnconnected=off
  wires:
  Abs/1 -> Relational Operator/1
  Abs(Vref)/1 -> Abs/1
  Ac7/1 -> Abs1/1
  Sum1/1 -> Relational Operator/2
  Abs1/1 -> Sum1/1
  Constant1/1 -> Sum1/2
  Relational Operator/1 -> Logical Operator/1
  Sum2/1 -> Relational Operator1/2
  Ac4/1 -> Abs3/1
  Constant2/1 -> Sum2/2
  Abs3/1 -> Sum2/1
  Abs(Vref)1/1 -> Abs2/1
  Abs2/1 -> Relational Operator1/1
  Relational Operator1/1 -> Logical Operator/2
  Logical Operator/1 -> Sp3/1

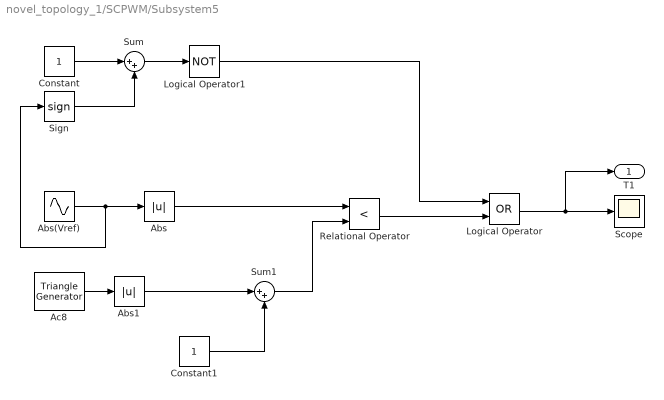
== system novel_topology_1/SCPWM/Subsystem5 ==
  Abs : Abs
  Abs(Vref) : Sin  Amplitude=ar  Frequency=2*pi*50  SampleTime=0
  Abs1 : Abs
  Ac8 : powerlib_meascontrol/Pulse & Signal Generators/Triangle Generator  Freq=cf  Phase=90  Ts=0
  Constant : Constant
  Constant1 : Constant
  Logical Operator : Logic  Operator=OR  AllPortsSameDT=off  OutDataTypeStr=boolean
  Logical Operator1 : Logic  Operator=NOT  AllPortsSameDT=off  OutDataTypeStr=boolean
  Relational Operator : RelationalOperator  Operator=<  OutDataTypeStr=boolean  RndMeth=Nearest
  Scope : Scope
  Sign : Signum
  Sum : Sum  Inputs=|++
  Sum1 : Sum  Inputs=|++
  T1 : Outport  VectorParamsAs1DForOutWhenUnconnected=off
  wires:
  Abs/1 -> Relational Operator/1
  Abs(Vref)/1 -> Sign/1, Abs/1
  Ac8/1 -> Abs1/1
  Sign/1 -> Sum/2
  Constant/1 -> Sum/1
  Sum1/1 -> Relational Operator/2
  Abs1/1 -> Sum1/1
  Constant1/1 -> Sum1/2
  Relational Operator/1 -> Logical Operator/2
  Sum/1 -> Logical Operator1/1
  Logical Operator/1 -> T1/1, Scope/1
  Logical Operator1/1 -> Logical Operator/1

== system novel_topology_1/SCPWM/Subsystem6 ==
  Abs : Abs
  Abs(Vref) : Sin  Amplitude=ar  Frequency=2*pi*50  SampleTime=0
  Abs1 : Abs
  Ac8 : powerlib_meascontrol/Pulse & Signal Generators/Triangle Generator  Freq=cf  Phase=90  Ts=0
  Constant : Constant
  Constant1 : Constant
  Logical Operator : Logic  Operator=OR  AllPortsSameDT=off  OutDataTypeStr=boolean
  Relational Operator : RelationalOperator  Operator=<  OutDataTypeStr=boolean  RndMeth=Nearest
  Scope : Scope
  Sign : Signum
  Sum : Sum  Inputs=|++
  Sum1 : Sum  Inputs=|++
  T2 : Outport  VectorParamsAs1DForOutWhenUnconnected=off
  wires:
  Abs/1 -> Relational Operator/1
  Abs(Vref)/1 -> Sign/1, Abs/1
  Ac8/1 -> Abs1/1
  Sign/1 -> Sum/2
  Constant/1 -> Sum/1
  Sum1/1 -> Relational Operator/2
  Abs1/1 -> Sum1/1
  Constant1/1 -> Sum1/2
  Relational Operator/1 -> Logical Operator/2
  Logical Operator/1 -> T2/1, Scope/1
  Sum/1 -> Logical Operator/1

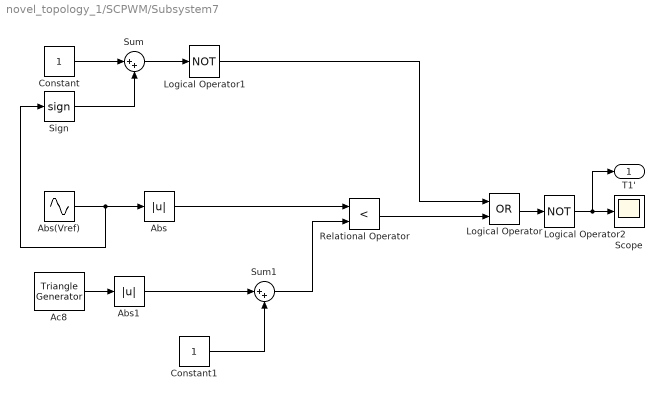
== system novel_topology_1/SCPWM/Subsystem7 ==
  Abs : Abs
  Abs(Vref) : Sin  Amplitude=ar  Frequency=2*pi*50  SampleTime=0
  Abs1 : Abs
  Ac8 : powerlib_meascontrol/Pulse & Signal Generators/Triangle Generator  Freq=cf  Phase=90  Ts=0
  Constant : Constant
  Constant1 : Constant
  Logical Operator : Logic  Operator=OR  AllPortsSameDT=off  OutDataTypeStr=boolean
  Logical Operator1 : Logic  Operator=NOT  AllPortsSameDT=off  OutDataTypeStr=boolean
  Logical Operator2 : Logic  Operator=NOT  AllPortsSameDT=off  OutDataTypeStr=boolean
  Relational Operator : RelationalOperator  Operator=<  OutDataTypeStr=boolean  RndMeth=Nearest
  Scope : Scope
  Sign : Signum
  Sum : Sum  Inputs=|++
  Sum1 : Sum  Inputs=|++
  T1' : Outport  VectorParamsAs1DForOutWhenUnconnected=off
  wires:
  Abs/1 -> Relational Operator/1
  Abs(Vref)/1 -> Sign/1, Abs/1
  Ac8/1 -> Abs1/1
  Sign/1 -> Sum/2
  Constant/1 -> Sum/1
  Sum1/1 -> Relational Operator/2
  Abs1/1 -> Sum1/1
  Constant1/1 -> Sum1/2
  Relational Operator/1 -> Logical Operator/2
  Sum/1 -> Logical Operator1/1
  Logical Operator/1 -> Logical Operator2/1
  Logical Operator1/1 -> Logical Operator/1
  Logical Operator2/1 -> T1'/1, Scope/1

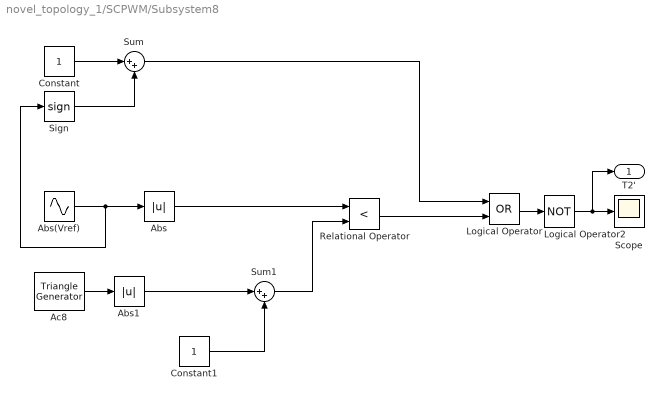
== system novel_topology_1/SCPWM/Subsystem8 ==
  Abs : Abs
  Abs(Vref) : Sin  Amplitude=ar  Frequency=2*pi*50  SampleTime=0
  Abs1 : Abs
  Ac8 : powerlib_meascontrol/Pulse & Signal Generators/Triangle Generator  Freq=cf  Phase=90  Ts=0
  Constant : Constant
  Constant1 : Constant
  Logical Operator : Logic  Operator=OR  AllPortsSameDT=off  OutDataTypeStr=boolean
  Logical Operator2 : Logic  Operator=NOT  AllPortsSameDT=off  OutDataTypeStr=boolean
  Relational Operator : RelationalOperator  Operator=<  OutDataTypeStr=boolean  RndMeth=Nearest
  Scope : Scope
  Sign : Signum
  Sum : Sum  Inputs=|++
  Sum1 : Sum  Inputs=|++
  T2' : Outport  VectorParamsAs1DForOutWhenUnconnected=off
  wires:
  Abs/1 -> Relational Operator/1
  Abs(Vref)/1 -> Sign/1, Abs/1
  Ac8/1 -> Abs1/1
  Sign/1 -> Sum/2
  Constant/1 -> Sum/1
  Sum1/1 -> Relational Operator/2
  Abs1/1 -> Sum1/1
  Constant1/1 -> Sum1/2
  Relational Operator/1 -> Logical Operator/2
  Logical Operator/1 -> Logical Operator2/1
  Sum/1 -> Logical Operator/1
  Logical Operator2/1 -> T2'/1, Scope/1
